simulink model "trajectory_optimization"  (R2014a)
settings: Solver=FixedStepDiscrete  StartTime=0.0  StopTime=inf  FixedStep=sample_time  RelTol=1e-3
undefined symbols (not defined in the file): alpha_apex, boom_mount_angle, control_start_time, d_y_boom_com_offset, d_y_boom_hip_offset, d_y_com, d_y_mount_to_com, DiscIntNeverNeededParam, g, h_boom, i_limit_lateral, j_segments, kd_angle, kd_lateral, kd_length, kd_motor, ki_lateral, kp_angle, kp_lateral, kp_length, kp_motor, l0_virtual, l_boom, l_boom_projected, l_retract_swing, l_seg, lateral_offset, m_leg_motor, magnitude, max_back_bar_angle, max_front_bar_angle, max_leg_angle, max_leg_length, max_torque_lateral, min_back_bar_angle, min_front_bar_angle, min_leg_angle, min_leg_length, reset_leg_angle, reset_leg_length, run_trajectory, sample_time, sea_coulomb_friction, sea_offset_friction, secondary_to_apex_target, time_to_apex, velocity_avg_samples
libraries: simulink x5
(part 2 of 2)

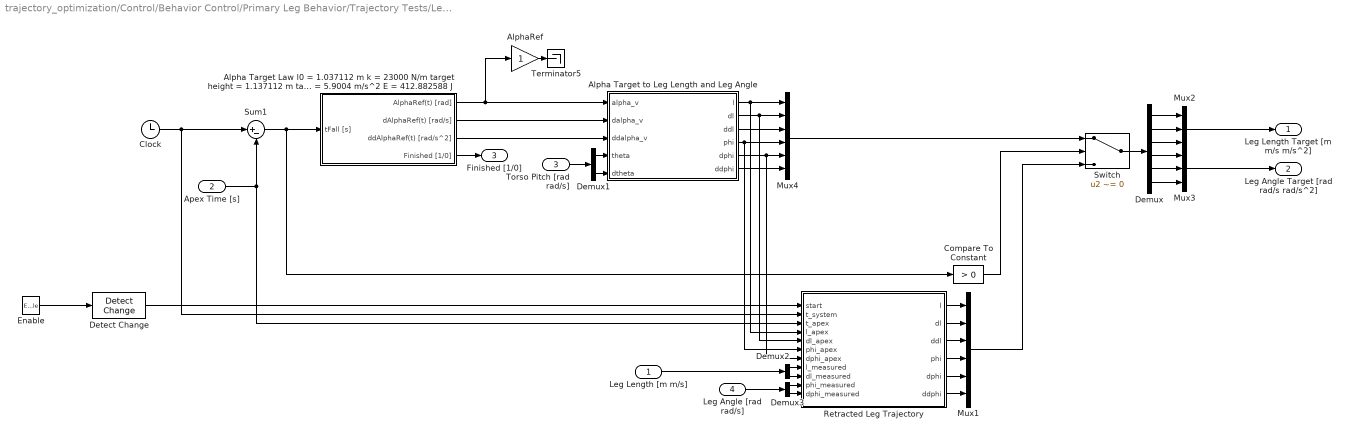
== system trajectory_optimization/Control/Behavior Control/Primary Leg Behavior/Trajectory Tests/Leg Trajectory Generator ==
  Leg Length [m m/s] : Inport
  Apex Time [s] : Inport  Port=2
  Torso Pitch [rad rad/s] : Inport  Port=3
  Leg Angle [rad rad/s] : Inport  Port=4
  Enable : EnablePort  StatesWhenEnabling=reset  ShowOutputPort=on  ZeroCross=off
      settings: AttributesFormatString=When enabled: %<StatesWhenEnabling>
  Alpha Target Law l0 = 1.037112 m k = 23000 N/m target height = 1.137112 m target speed = 0.5 m/s m = 60.4120 kg g = 5.9004 m/s^2 E = 412.882588 J : Subsystem
  Alpha Target to Leg Length and Leg Angle : MATLAB Function  TreatAsAtomicUnit=on
  AlphaRef : Gain
  Clock : Clock
  Compare To Constant : simulink/Logic and Bit Operations/Compare To Constant  relop=>  const=0  OutDataTypeStr=boolean  ZeroCross=off
  Demux : Demux  Outputs=6
  Demux1 : Demux  Outputs=2
  Demux2 : Demux  Outputs=2
  Demux3 : Demux  Outputs=2
  Detect Change : simulink/Logic and Bit Operations/Detect Change  vinit=0  InputProcessing=Inherited  OutDataTypeStr=boolean
  Mux1 : Mux  Inputs=6
  Mux2 : Mux  Inputs=3
  Mux3 : Mux  Inputs=3
  Mux4 : Mux  Inputs=6
  Retracted Leg Trajectory : MATLAB Function  TreatAsAtomicUnit=on
  Sum1 : Sum  Inputs=|+-
  Switch : Switch  Criteria=u2 ~= 0
  Terminator5 : Terminator
  Leg Length Target [m m/s m/s^2] : Outport
  Leg Angle Target [rad rad/s rad/s^2] : Outport  Port=2
  Finished [1/0] : Outport  Port=3  OutDataTypeStr=boolean
  wires:
  Torso Pitch [rad rad/s]/1 -> Demux1/1
  Mux1/1 -> Switch/3
  Compare To Constant/1 -> Switch/2
  Apex Time [s]/1 -> Retracted Leg Trajectory/3(t_apex), Sum1/2
  Clock/1 -> Retracted Leg Trajectory/2(t_system), Sum1/1
  Alpha Target Law l0 = 1.037112 m k = 23000 N/m target height = 1.137112 m target speed = 0.5 m/s m = 60.4120 kg g = 5.9004 m/s^2 E = 412.882588 J/1(AlphaRef(t) [rad]) -> AlphaRef/1, Alpha Target to Leg Length and Leg Angle/1(alpha_v)
  Sum1/1 -> Compare To Constant/1, Alpha Target Law l0 = 1.037112 m k = 23000 N/m target height = 1.137112 m target speed = 0.5 m/s m = 60.4120 kg g = 5.9004 m/s^2 E = 412.882588 J/1(tFall [s])
  AlphaRef/1 -> Terminator5/1
  Alpha Target Law l0 = 1.037112 m k = 23000 N/m target height = 1.137112 m target speed = 0.5 m/s m = 60.4120 kg g = 5.9004 m/s^2 E = 412.882588 J/4(Finished [1/0]) -> Finished [1/0]/1
  Retracted Leg Trajectory/1(l) -> Mux1/1
  Retracted Leg Trajectory/4(phi) -> Mux1/4
  Retracted Leg Trajectory/2(dl) -> Mux1/2
  Retracted Leg Trajectory/5(dphi) -> Mux1/5
  Enable/1 -> Detect Change/1
  Detect Change/1 -> Retracted Leg Trajectory/1(start)
  Alpha Target to Leg Length and Leg Angle/4(phi) -> Retracted Leg Trajectory/6(phi_apex), Mux4/4
  Alpha Target to Leg Length and Leg Angle/3(ddl) -> Mux4/3
  Alpha Target to Leg Length and Leg Angle/5(dphi) -> Retracted Leg Trajectory/7(dphi_apex), Mux4/5
  Alpha Target to Leg Length and Leg Angle/6(ddphi) -> Mux4/6
  Alpha Target to Leg Length and Leg Angle/2(dl) -> Retracted Leg Trajectory/5(dl_apex), Mux4/2
  Alpha Target to Leg Length and Leg Angle/1(l) -> Retracted Leg Trajectory/4(l_apex), Mux4/1
  Switch/1 -> Demux/1
  Mux2/1 -> Leg Length Target [m m/s m/s^2]/1
  Mux3/1 -> Leg Angle Target [rad rad/s rad/s^2]/1
  Demux/6 -> Mux3/3
  Demux/5 -> Mux3/2
  Demux/4 -> Mux3/1
  Demux/3 -> Mux2/3
  Demux/2 -> Mux2/2
  Demux/1 -> Mux2/1
  Demux1/1 -> Alpha Target to Leg Length and Leg Angle/4(theta)
  Demux1/2 -> Alpha Target to Leg Length and Leg Angle/5(dtheta)
  Mux4/1 -> Switch/1
  Alpha Target Law l0 = 1.037112 m k = 23000 N/m target height = 1.137112 m target speed = 0.5 m/s m = 60.4120 kg g = 5.9004 m/s^2 E = 412.882588 J/3(ddAlphaRef(t) [rad/s^2]) -> Alpha Target to Leg Length and Leg Angle/3(ddalpha_v)
  Alpha Target Law l0 = 1.037112 m k = 23000 N/m target height = 1.137112 m target speed = 0.5 m/s m = 60.4120 kg g = 5.9004 m/s^2 E = 412.882588 J/2(dAlphaRef(t) [rad/s]) -> Alpha Target to Leg Length and Leg Angle/2(dalpha_v)
  Retracted Leg Trajectory/3(ddl) -> Mux1/3
  Retracted Leg Trajectory/6(ddphi) -> Mux1/6
  Demux2/1 -> Retracted Leg Trajectory/8(l_measured)
  Demux2/2 -> Retracted Leg Trajectory/9(dl_measured)
  Demux3/1 -> Retracted Leg Trajectory/10(phi_measured)
  Demux3/2 -> Retracted Leg Trajectory/11(dphi_measured)
  Leg Angle [rad rad/s]/1 -> Demux3/1
  Leg Length [m m/s]/1 -> Demux2/1

== system trajectory_optimization/Control/Behavior Control/Primary Leg Behavior/Trajectory Tests/Saturations ==
  "[l dl ddl phi dphi ddphi]" : Inport
  Demux3 : Demux  Outputs=6
  Leg Angle Limits : Saturate  UpperLimit=max_leg_angle  LowerLimit=min_leg_angle
      settings: AttributesFormatString=Hi: %<UpperLimit>\nLo: %<LowerLimit>
  Leg Length Limits : Saturate  UpperLimit=max_leg_length  LowerLimit=min_leg_length
      settings: AttributesFormatString=Hi: %<UpperLimit>\nLo: %<LowerLimit>
  Mux5 : Mux  Inputs=6
  limited : Outport
  wires:
  Mux5/1 -> limited/1
  "[l dl ddl phi dphi ddphi]"/1 -> Demux3/1
  Demux3/4 -> Leg Angle Limits/1
  Demux3/1 -> Leg Length Limits/1
  Leg Length Limits/1 -> Mux5/1
  Demux3/2 -> Mux5/2
  Leg Angle Limits/1 -> Mux5/4
  Demux3/5 -> Mux5/5
  Demux3/3 -> Mux5/3
  Demux3/6 -> Mux5/6

== system trajectory_optimization/Control/Behavior Control/Primary Leg Behavior/Trajectory Tests/Tracking Errors ==
  Error 1 : Inport
  Error 2 : Inport  Port=2
  Enable : EnablePort  ShowOutputPort=on
  AngleError : DiscreteIntegrator  IntegratorMethod=Accumulation: Forward Euler  gainval=sample_time  ExternalReset=rising  SampleTime=sample_time  ICPrevOutput=DiscIntNeverNeededParam  ICPrevScaledInput=DiscIntNeverNeededParam
  LengthError : DiscreteIntegrator  IntegratorMethod=Accumulation: Forward Euler  gainval=sample_time  ExternalReset=rising  SampleTime=sample_time  ICPrevOutput=DiscIntNeverNeededParam  ICPrevScaledInput=DiscIntNeverNeededParam
  Math Function : Math  Operator=magnitude^2  SaturateOnIntegerOverflow=on
  Math Function1 : Math  Operator=magnitude^2  SaturateOnIntegerOverflow=on
  Sum : Sum  Inputs=+|+
  Error Sum 1 : Outport  InitialOutput=0
  Error Sum 2 : Outport  Port=2  InitialOutput=0
  Total Error : Outport  Port=3  InitialOutput=0
  wires:
  Math Function/1 -> LengthError/1
  Math Function1/1 -> AngleError/1
  Error 2/1 -> Math Function1/1
  AngleError/1 -> Error Sum 2/1, Sum/2
  LengthError/1 -> Error Sum 1/1, Sum/1
  Error 1/1 -> Math Function/1
  Enable/1 -> LengthError/2, AngleError/2
  Sum/1 -> Total Error/1

== system trajectory_optimization/Control/Behavior Control/Secondary Leg Behavior/Back//Front Motor PD/Friction Compensation ==
  Right/Left [1/0] : Inport
  Commanded Velocity [rad/s] [back front] : Inport  Port=2
  Product : Product
  Sign : Signum
  Sum1 : Sum
  Switch : Switch  Criteria=u2 ~= 0
  Switch1 : Switch  Criteria=u2 ~= 0
  coulomb_friction_left : Constant  Value=sea_coulomb_friction(3:4)
  coulomb_friction_right : Constant  Value=sea_coulomb_friction(1:2)
  offset_friction_left : Constant  Value=sea_offset_friction(3:4)
  offset_friction_right : Constant  Value=sea_offset_friction(1:2)
  Friction Compensation [Nm] : Outport
  wires:
  Commanded Velocity [rad/s] [back front]/1 -> Sign/1
  Switch/1 -> Sum1/2
  Sum1/1 -> Friction Compensation [Nm]/1
  Product/1 -> Sum1/1
  Right/Left [1/0]/1 -> Switch1/2, Switch/2
  offset_friction_right/1 -> Switch/1
  offset_friction_left/1 -> Switch/3
  coulomb_friction_right/1 -> Switch1/1
  coulomb_friction_left/1 -> Switch1/3
  Switch1/1 -> Product/2
  Sign/1 -> Product/1

== system trajectory_optimization/Control/Behavior Control/Primary Leg Behavior/Trajectory Tests/Back Motor PD/Friction Compensation ==
  Commanded Velocity [rad/s] : Inport
  Constant1 : Constant  Value=sea_offset_friction(1)
  KdGain2 : Gain  Description=xPCTag(1)=kd_sea_torque;  Gain=sea_coulomb_friction(1)
  Sign : Signum
  Sum1 : Sum
  Friction Compensation [Nm] : Outport
  wires:
  Sign/1 -> KdGain2/1
  Commanded Velocity [rad/s]/1 -> Sign/1
  Constant1/1 -> Sum1/2
  Sum1/1 -> Friction Compensation [Nm]/1
  KdGain2/1 -> Sum1/1

== system trajectory_optimization/Control/Behavior Control/Primary Leg Behavior/Trajectory Tests/Front Motor PD/Friction Compensation ==
  Commanded Velocity [rad/s] : Inport
  Constant1 : Constant  Value=sea_offset_friction(2)
  KdGain2 : Gain  Description=xPCTag(1)=kd_sea_torque;  Gain=sea_coulomb_friction(2)
  Sign : Signum
  Sum1 : Sum
  Friction Compensation [Nm] : Outport
  wires:
  Sign/1 -> KdGain2/1
  Commanded Velocity [rad/s]/1 -> Sign/1
  Constant1/1 -> Sum1/2
  Sum1/1 -> Friction Compensation [Nm]/1
  KdGain2/1 -> Sum1/1

== system trajectory_optimization/Control/Behavior Control/Primary Leg Behavior/Trajectory Tests/Leg Trajectory Generator/Alpha Target Law l0 = 1.037112 m k = 23000 N//m target height = 1.137112 m target speed = 0.5 m//s m = 60.4120 kg g = 5.9004 m//s^2 E = 412.882588 J ==
  note: Angle of Attack Control Law From Poincare Map Method
  tFall [s] : Inport
  Alpha Target Polynomials : Subsystem
  AlphaRef1 : Constant  Value=[(90+20)*pi/180 0 0]
  Compare To Constant1 : simulink/Logic and Bit Operations/Compare To Constant  relop=<  const=0.2464038  OutDataTypeStr=boolean  ZeroCross=off
  Demux : Demux  Outputs=3
  Ignore Negatives : Fcn  Expr=(u >= 0)*u
  Logical Operator : Logic  Operator=NOT  AllPortsSameDT=off  OutDataTypeStr=boolean
  Mux : Mux  Inputs=3
  Switch : Switch  Criteria=u2 ~= 0
  AlphaRef(t) [rad] : Outport
  dAlphaRef(t) [rad/s] : Outport  Port=2
  ddAlphaRef(t) [rad/s^2] : Outport  Port=3
  Finished [1/0] : Outport  Port=4  OutDataTypeStr=boolean
  wires:
  AlphaRef1/1 -> Switch/3
  Demux/3 -> ddAlphaRef(t) [rad/s^2]/1
  Demux/2 -> dAlphaRef(t) [rad/s]/1
  Demux/1 -> AlphaRef(t) [rad]/1
  Switch/1 -> Demux/1
  tFall [s]/1 -> Ignore Negatives/1, Compare To Constant1/1
  Compare To Constant1/1 -> Logical Operator/1, Switch/2
  Logical Operator/1 -> Finished [1/0]/1
  Alpha Target Polynomials/2(dAlphaRef(t)) -> Mux/2
  Alpha Target Polynomials/3(ddAlphaRef(t)) -> Mux/3
  Alpha Target Polynomials/1(AlphaRef(t)) -> Mux/1
  Mux/1 -> Switch/1
  Ignore Negatives/1 -> Alpha Target Polynomials/1(tFall)

== system trajectory_optimization/Control/Behavior Control/Primary Leg Behavior/Trajectory Tests/Leg Trajectory Generator/Alpha Target Law l0 = 1.037112 m k = 23000 N//m target height = 1.137112 m target speed = 0.5 m//s m = 60.4120 kg g = 5.9004 m//s^2 E = 412.882588 J/Alpha Target Polynomials ==
  tFall : Inport
  AlphaRef(t) Control Law : Fcn  Expr=18.34*u^3 + 4.673*u^2 + 1.844*u + alpha_apex
  acceleration of AlphaRef(t) Control Law : Fcn  Expr=2*3*18.34*u + 2*4.673
  velocity of AlphaRef(t) Control Law : Fcn  Expr=3*18.34*u^2 + 2*4.673*u + 1.844
  AlphaRef(t) : Outport  OutputWhenDisabled=reset  InitialOutput=0
      settings: AttributesFormatString=When disabled: %<OutputWhenDisabled>\nDisabled Output: %<InitialOutput>
  dAlphaRef(t) : Outport  Port=2  OutputWhenDisabled=reset  InitialOutput=0
      settings: AttributesFormatString=When disbaled: %<OutputWhenDisabled>\nDisabled output: %<InitialOutput>
  ddAlphaRef(t) : Outport  Port=3  OutputWhenDisabled=reset  InitialOutput=0
      settings: AttributesFormatString=When disabled: %<OutputWhenDisabled>\nDisabled output: %<InitialOutput>
  wires:
  acceleration of AlphaRef(t) Control Law/1 -> ddAlphaRef(t)/1
  velocity of AlphaRef(t) Control Law/1 -> dAlphaRef(t)/1
  AlphaRef(t) Control Law/1 -> AlphaRef(t)/1
  tFall/1 -> acceleration of AlphaRef(t) Control Law/1, velocity of AlphaRef(t) Control Law/1, AlphaRef(t) Control Law/1

== matlab function trajectory_optimization/Control/Behavior Control/Primary Leg Behavior/Trajectory Tests/Leg Trajectory Generator/Retracted Leg Trajectory ==
  data: start input; t_system input; t_apex input; l_apex input; dl_apex input; phi_apex input; dphi_apex input; l_measured input; dl_measured input; phi_measured input; l output; dl output; ddl output; phi output; dphi output; ddphi output; dphi_measured input
%% Generates a dynamically feasible trajectory for swinging the virtual leg between two points.
% Constrains to starting/ending positions and velocities.
% Minimizes torque squared
% May want to generate the trajectory in fourbar coordinates instead.
function [l, dl, ddl, phi, dphi, ddphi] = fcn(start, t_system, t_apex, l_apex, dl_apex, phi_apex, dphi_apex, l_measured, dl_measured, phi_measured, dphi_measured)

    persistent t_start l_start phi_start dl_start dphi_start;
    if isempty(t_start) || start
        t_start = t_system;
        l_start = l_measured;
        dl_start = dl_measured;
        phi_start = phi_measured;
        dphi_start = dphi_measured;
    end
    
    t = t_system - t_start;
    time_to_apex = t_apex - t_start;
    t = min(time_to_apex, t);

    % Virtual Leg Length
    [a0, a1, a2, a3] = ThirdOrderTrajectory(l_start, dl_start, l_apex, dl_apex, time_to_apex);
    l = a3*t^3 + a2*t^2 + a1*t + a0;
    dl = 3*a3*t^2 + 2*a2*t + a1;
    ddl = 6*a3*t + 2*a2;
    
    % Virtual Leg Angle
    [a0, a1, a2, a3] = ThirdOrderTrajectory(phi_start, dphi_start, phi_apex, dphi_apex, time_to_apex);
    phi = a3*t^3 + a2*t^2 + a1*t + a0;
    dphi = 3*a3*t^2 + 2*a2*t + a1;
    ddphi = 6*a3*t + 2*a2;

end

== matlab function trajectory_optimization/Control/Behavior Control/Secondary Leg Behavior/Virtual Leg to Four Bar ==
  data: l_leg input; dl_leg input; ddl_leg input; phi input; dphi input; ddphi input; back output; dback output; ddback output; front output; dfront output; ddfront output
function [back, dback, ddback, front, dfront, ddfront] = fcn(l_leg, dl_leg, ddl_leg, phi, dphi, ddphi)
    [back, dback, ddback, front, dfront, ddfront] = VirtualLegToFourBar(l_leg, dl_leg, ddl_leg, phi, dphi, ddphi);
end

== matlab function trajectory_optimization/Control/Behavior Control/Secondary Leg Behavior/Virtual Leg Trajectory Towards Alpha Apex Target ==
  data: start input; t_system input; l_leg output; dl_leg output; ddl_leg output; phi output; dphi output; ddphi output; alpha_apex parameter; theta input; l_measured input; dl_measured input; phi_measured input; dphi_measured input; d_y_com parameter; l0_virtual parameter
%% Create a trajectory between starting position/velocity and some alpha
% The goal is to move the system towards the alpha target at apex.
function [l_leg, dl_leg, ddl_leg, phi, dphi, ddphi] = fcn(start, t_system, alpha_apex, theta, l_measured, dl_measured, phi_measured, dphi_measured, d_y_com, l0_virtual)
    % Should the target be less than apex position? midpoint?
    [l_apex, dl_apex, ~, phi_apex, dphi_apex, ~] = AlphaTargetToVirtualLeg2D(alpha_apex, 0, 0, theta, 0, 0, d_y_com, l0_virtual);
    
    persistent t_start l_start phi_start dl_start dphi_start;
    if isempty(t_start) || start
        t_start = t_system;
        l_start = l_measured;
        dl_start = dl_measured;
        phi_start = phi_measured;
        dphi_start = dphi_measured;
    end
    

    time_to_takeoff = 0.400;  % Overestimate, How to approximate this?
    t = t_system - t_start;
    t = min(time_to_takeoff, t);
    
    % Virtual Leg Length
    [a0, a1, a2, a3] = ThirdOrderTrajectory(l_start, dl_start, l_apex, dl_apex, time_to_takeoff);
    l_leg = a3*t^3 + a2*t^2 + a1*t + a0;
    dl_leg = 3*a3*t^2 + 2*a2*t + a1;
    ddl_leg = 6*a3*t + 2*a2;
    
    % Virtual Leg Angle
    [a0, a1, a2, a3] = ThirdOrderTrajectory(phi_start, dphi_start, phi_apex, dphi_apex, time_to_takeoff);
    phi = a3*t^3 + a2*t^2 + a1*t + a0;
    dphi = 3*a3*t^2 + 2*a2*t + a1;
    ddphi = 6*a3*t + 2*a2;
end

== matlab function trajectory_optimization/Control/Behavior Control/Primary Leg Behavior/Trajectory Tests/Leg Trajectory Generator/Alpha Target to Leg Length and Leg Angle ==
  data: alpha_v input; dalpha_v input; ddalpha_v input; theta input; dtheta input; l output; dl output; ddl output; phi output; d_y_com parameter; l0_virtual parameter; dphi output; ddphi output
function [l, dl, ddl, phi, dphi, ddphi] = fcn(alpha_v, dalpha_v, ddalpha_v, theta, dtheta, d_y_com, l0_virtual)
    [l, dl, ddl, phi, dphi, ddphi] = AlphaTargetToVirtualLeg2D(alpha_v, dalpha_v, ddalpha_v, theta, dtheta, 0, d_y_com, l0_virtual);
end

== matlab function trajectory_optimization/Control/Behavior Control/Primary Leg Behavior/Trajectory Tests/Virtual Leg to Four Bar ==
  data: phi input; dphi input; ddphi input; l_leg input; dl_leg input; back output; dback output; ddback output; front output; dfront output; ddl_leg input; ddfront output
function [back, dback, ddback, front, dfront, ddfront] = fcn(phi, dphi, ddphi, l_leg, dl_leg, ddl_leg)   
    [back, dback, ddback, front, dfront, ddfront] = VirtualLegToFourBar(l_leg, dl_leg, ddl_leg, phi, dphi, ddphi);
end

== matlab function trajectory_optimization/Control/Behavior Control/Velocity Estimation/dx_and_dy_from_yaw_and_roll ==
  data: qRoll input; dqRoll input; dx output; dqYaw input; dqPitch input; l_boom parameter; l_boom_projected parameter; h_boom parameter; boom_mount_angle parameter; d_y_boom_com_offset parameter; d_y_boom_hip_offset parameter; dy output; d_y_mount_to_com parameter; y_com output; y_hip output
function [dx, dy, y_com, y_hip] = fcn(qRoll, dqRoll, dqYaw, dqPitch, ...
                        l_boom, l_boom_projected, h_boom, boom_mount_angle, ...
                        d_y_boom_com_offset, d_y_boom_hip_offset, d_y_mount_to_com)
    % dx
    x_boom = l_boom * cos(qRoll);
    x_mount_to_center = d_y_mount_to_com * sin(qRoll-boom_mount_angle);
    dx = dqYaw * (x_boom + x_mount_to_center) - dqPitch * d_y_mount_to_com;
    
    % dy
    dy    = dqRoll * l_boom_projected * cos(qRoll)  +  d_y_boom_com_offset * dqRoll * sin(qRoll-boom_mount_angle);
    
    % y (COM and hip point)
    y_com = h_boom + l_boom_projected * sin(qRoll)  -  d_y_boom_com_offset * cos(qRoll-boom_mount_angle); 
    y_hip = h_boom + l_boom_projected * sin(qRoll)  -  d_y_boom_hip_offset * cos(qRoll-boom_mount_angle); 
end

== matlab function trajectory_optimization/Control/Behavior Control/Virtual Spring Calculator/Virtual Spring Calculations ==
  data: th input; alpha_v output; dth input; l input; dl input; phi input; dphi input; dalpha_v output; l_v output; dl_v output; d_y_com parameter
function [alpha_v, dalpha_v, l_v, dl_v] = fcn(th, dth, l, dl, phi, dphi, d_y_com)

gma = th + phi;
dgma = dth + dphi;
d = d_y_com;

xf  =  l*sin(gma) - d*sin(th);
dxf =  l*dgma*cos(gma) + dl*sin(gma) - d*dth*cos(th);
yf  = -l*cos(gma) + d*cos(th);
dyf =  l*dgma*sin(gma) - dl*cos(gma) - d*dth*sin(th);

alpha_v  = atan2(yf, xf);
dalpha_v = 1/(1+(yf/xf)^2) * (xf*dyf - yf*dxf)/xf^2;

l_v  = (d^2 + l^2 - 2*d*l*cos(phi))^0.5;
dl_v = (l*dl - d*dl*cos(phi) + d*l*dphi*sin(phi))/l_v;

end

== matlab function trajectory_optimization/Control/Behavior Control/Secondary Leg Behavior/Avoid Hitting Mechanical Limits ==
  data: back_cmd output; front_cmd output; dback_cmd output; dfront_cmd output; ddback_cmd output; ddfront_cmd output; back_desired input; dback_desired input; ddback_desired input; front_desired input; dfront_desired input; ddfront_desired input; min_front_bar_angle parameter; max_front_bar_angle parameter; min_back_bar_angle parameter; max_back_bar_angle parameter
%% Avoid joint limits by ensuring we don't command velocities/accelerations that would push us into them when we are close to them.
function [back_cmd, front_cmd, dback_cmd, dfront_cmd, ddback_cmd, ddfront_cmd] ...
    = fcn(back_desired,dback_desired, ddback_desired, ...
          front_desired, dfront_desired, ddfront_desired, ...
          min_front_bar_angle, max_front_bar_angle, min_back_bar_angle, max_back_bar_angle)

    min_back_distance = back_desired - min_back_bar_angle;
    max_back_distance = max_back_bar_angle - back_desired;
    min_front_distance = front_desired - min_front_bar_angle;
    max_front_distance = max_front_bar_angle - front_desired;

    back_cmd = min(max(back_desired, min_back_bar_angle), max_back_bar_angle);
    front_cmd = min(max(front_desired, min_front_bar_angle), max_front_bar_angle);
    dback_cmd = dback_desired;
    dfront_cmd = dfront_desired;
    ddback_cmd = ddback_desired;
    ddfront_cmd = ddfront_desired;

    distance_threshold = 10*pi/180;

    if (min_back_distance < distance_threshold && sign(dback_desired) < 0) || ...
       (max_back_distance < distance_threshold && sign(dback_desired) > 0)
        dback_cmd = 0;
    end
    
    if (min_back_distance < distance_threshold && sign(ddback_desired) < 0) || ...
       (max_back_distance < distance_threshold && sign(ddback_desired) > 0)
        ddback_cmd = 0;
    end

    if (min_front_distance < distance_threshold && sign(dfront_desired) < 0) || ...
       (max_front_distance < distance_threshold && sign(dfront_desired) > 0)
        dfront_cmd = 0;
    end
    
    if (min_front_distance < distance_threshold && sign(ddfront_desired) < 0) || ...
       (max_front_distance < distance_threshold && sign(ddfront_desired) > 0)
        ddfront_cmd = 0;
    end

end
